simulink model "compare_sim"  (R2020b)
settings: Solver=VariableStepAuto  StartTime=0.0  StopTime=time(end)  RelTol=1e-3
values from neighbouring files (symbols this model uses):
  Cy = 27229.08    [compare_data.m]
  Jz = 2393.665    [LoadVehicleParameters.m]    (also in compare_data.m)
  lf = 1.311    [LoadVehicleParameters.m]    (also in compare_data.m)
  lr = 1.311    [LoadVehicleParameters.m]    (also in compare_data.m)
  m = 1599.98    [LoadVehicleParameters.m]    (also in compare_data.m)
  Ts = 0.05    [compare_data.m]    (also in nl_identification.m = 0)
  Vx = u_ext(3)    [VehicleModelLTV.m]    (also in compare_data.m = 80)
  X = err_data.signals.values    [compare_data.m]
settings Model: Creator=LAMES Workstation  LastModifiedBy=LAMES Workstation

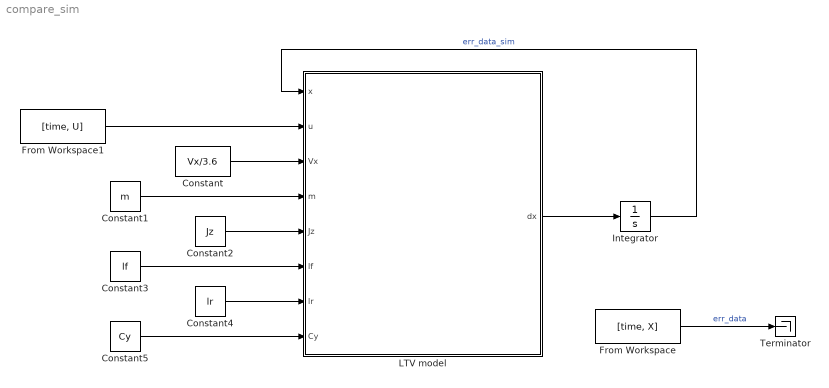
== system compare_sim ==
  Constant : Constant  Value=Vx/3.6
  Constant1 : Constant  Value=m
  Constant2 : Constant  Value=Jz
  Constant3 : Constant  Value=lf
  Constant4 : Constant  Value=lr
  Constant5 : Constant  Value=Cy
  From Workspace : FromWorkspace  VariableName=[time, X]  SampleTime=Ts
  From Workspace1 : FromWorkspace  VariableName=[time, U]  SampleTime=Ts
  Integrator : Integrator  InitialCondition=X(1,:)'
  LTV model : MATLAB Function  TreatAsAtomicUnit=on
  Terminator : Terminator
  wires:
  LTV model/1(dx) -> Integrator/1
  Integrator/1 -> LTV model/1(x)  "err_data_sim"
  From Workspace1/1 -> LTV model/2(u)
  Constant/1 -> LTV model/3(Vx)
  Constant1/1 -> LTV model/4(m)
  Constant2/1 -> LTV model/5(Jz)
  Constant3/1 -> LTV model/6(lf)
  Constant4/1 -> LTV model/7(lr)
  Constant5/1 -> LTV model/8(Cy)
  From Workspace/1 -> Terminator/1  "err_data"

== matlab function compare_sim/LTV model ==
  data: dx output; x input; u input; Vx input; m input; Jz input; lf input; lr input; Cy input
function dx = VehicleModelLTV(x,u,Vx,m,Jz,lf,lr,Cy)

    Cf = Cy;
    Cr = Cy;

    A = [0, 1, 0, 0;
        0, -(2*Cf+2*Cr)/m/Vx, (2*Cf+2*Cr)/m, -(2*Cf*lf-2*Cr*lr)/m/Vx;
        0, 0, 0, 1;
        0, -(2*Cf*lf-2*Cr*lr)/Jz/Vx, (2*Cf*lf-2*Cr*lr)/Jz, -(2*Cf*lf^2+2*Cr*lr^2)/Jz/Vx];
    B = [0, 2*Cf/m, 0, 2*Cf*lf/Jz]';
    B1 = [0, -(2*Cf*lf-2*Cr*lr)/m/Vx-Vx, 0, -(2*Cf*lf^2+2*Cr*lr^2)/Jz/Vx]';
    
    dx = A*x + [B/13,B1]*u;
    
end
